simulink model "agws_fastTT"  (R2016a)
settings: Solver=ode4  StartTime=0.0  StopTime=1  FixedStep=Ts  RelTol=1e-3
values from neighbouring files (symbols this model uses):
  M1_BeMo_d = zeros(7,M1_n_mode)    [AcO_Ctrl_headless_cfg.m]    (also in agws_cfg.m = 1e-6*bsxfun(@times,randn(7,M1_n_mode),scale); agws_fastTT_cfg.m = 1e-6*bsxfun(@times,randn(7,M1_n_mode),scale))
  M1_RiBo_d = zeros(7,6)    [AcO_Ctrl_headless_cfg.m]    (also in agws_cfg.m = [M1_Txyz0 M1_Rxyz0]; agws_fastTT_cfg.m = [M1_Txyz0 M1_Rxyz0])
  M2_RiBo_d = zeros(7,6)    [AcO_Ctrl_headless_cfg.m]    (also in agws_cfg.m = [M2_Txyz0 M2_Rxyz0]; agws_fastTT_cfg.m = [M2_Txyz0 M2_Rxyz0])
  Ts = 1/fs    (= 0.002)    [AcO_Ctrl_headless_cfg.m]    (also in agws_fastTT_cfg.m = 0.005)
undefined symbols (not defined in the file or in its folder): R
libraries: CEO x4
settings Model: Creator=rconan  LastModifiedBy=rconan
settings DataIOCC: LimitDataPoints=on  SaveFormat=Array
settings HardwareCC: ProdBitPerPointer=32  ProdLargestAtomicFloat=None  ProdIntDivRoundTo=Undefined  ProdEndianess=Unspecified  ProdWordSize=32  ProdHWDeviceType=32-bit Generic
settings ModelReferenceCC: PropagateSignalLabelsOutOfModel=off
settings ConfigComp: CovModelRefEnable=Off

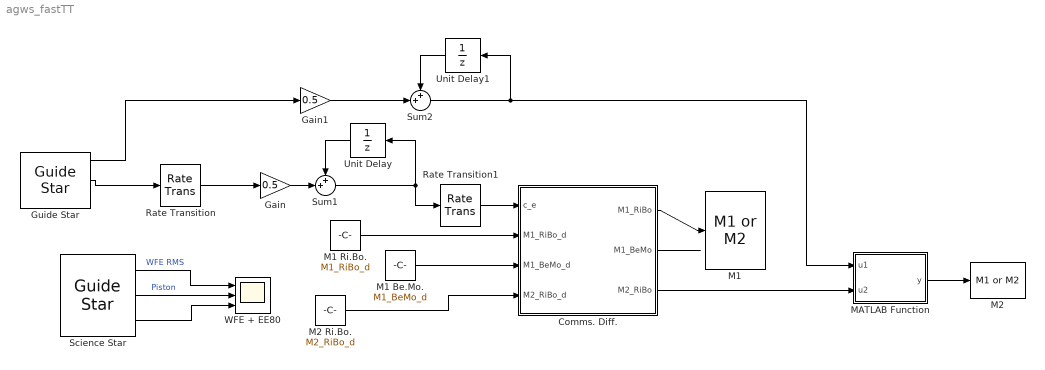
== system agws_fastTT ==
  Comms. Diff. : MATLAB Function  TreatAsAtomicUnit=on
  Gain : Gain  Gain=0.5
  Gain1 : Gain  Gain=0.5
  Guide Star : CEO/Guide Star  zenith=gs_zen  azimuth=gs_azi  photometry=R - 0.640  magnitude=0  rays_origin=[0,0,25]  rays_box_size=25.5  rays_box_sampling=16  sensor=GeometricShackHartmann  sampleTime=[Ts,0]  n_lenslet=30  d=26/30  n_cam=128  px_scale=NaN  intensity_threshold=0.2  a=1  b=1  wfe_rms=off  piston=off  segment_piston=off  ee80=off  sens=off  calibration_file=[upper(gcs),'_Calibration']  coms=gs_calib  coms_size=gs_calib_size  svd_truncation=[0,6]
  M1 : CEO/M1 or M2  mirror=M1  TxyzRxyz=on  mode_coefs=on  n_mode=42  sampleTime=[-1,0]
  M1 Be.Mo. : Constant  Value=M1_BeMo_d
  M1 Ri.Bo. : Constant  Value=M1_RiBo_d
  M2 : CEO/M1 or M2  mirror=M2  TxyzRxyz=on  mode_coefs=off  n_mode=66  sampleTime=[-1,0]
  M2 Ri.Bo. : Constant  Value=M2_RiBo_d
  MATLAB Function : MATLAB Function  TreatAsAtomicUnit=on
  Rate Transition : RateTransition  OutPortSampleTime=M1_Ts
  Rate Transition1 : RateTransition  OutPortSampleTime=Ts
  Science Star : CEO/Guide Star  zenith=0  azimuth=0  photometry=R - 0.640  magnitude=0  rays_origin=[0,0,25]  rays_box_size=25.5  rays_box_sampling=256  sensor=Imaging  sampleTime=[Ts,0]  n_lenslet=1  d=26  n_cam=128  px_scale=0.00127  intensity_threshold=0.5  a=2  b=1  wfe_rms=on  piston=off  segment_piston=on  ee80=on  sens=off  calibration_file=[]  coms=[]  coms_size=14  svd_truncation=0
  Sum1 : Sum  Inputs=++|
  Sum2 : Sum  Inputs=++|
  Unit Delay : UnitDelay  SampleTime=-1
  Unit Delay1 : UnitDelay  SampleTime=-1
  WFE + EE80 : Scope  NumInputPorts=3
  wires:
  Gain/1 -> Sum1/2
  Sum1/1 -> Rate Transition1/1, Unit Delay/1
  Unit Delay/1 -> Sum1/1
  Science Star/1 -> WFE + EE80/1  "WFE RMS"
  M1 Ri.Bo./1 -> Comms. Diff./2(M1_RiBo_d)
  Comms. Diff./1(M1_RiBo) -> M1/1
  Science Star/2 -> WFE + EE80/2  "Piston"
  Science Star/3 -> WFE + EE80/3
  Comms. Diff./2(M1_BeMo) -> ?
  M2 Ri.Bo./1 -> Comms. Diff./4(M2_RiBo_d)
  M1 Be.Mo./1 -> Comms. Diff./3(M1_BeMo_d)
  Guide Star/2 -> Rate Transition/1
  Rate Transition/1 -> Gain/1
  Rate Transition1/1 -> Comms. Diff./1(c_e)
  Gain1/1 -> Sum2/2
  Sum2/1 -> MATLAB Function/1(u1), Unit Delay1/1
  Unit Delay1/1 -> Sum2/1
  Guide Star/1 -> Gain1/1
  Comms. Diff./3(M2_RiBo) -> MATLAB Function/2(u2)
  MATLAB Function/1(y) -> M2/1

== matlab function agws_fastTT/MATLAB Function ==
  data: u1 input; y output; u2 input
function y = removeTT(u1,u2)
%#codegen

y = u2;
y(:,4:5) = u2(:,4:5) - reshape(u1,2,7)';

== matlab function agws_fastTT/Comms. Diff. ==
  data: c_e input; M1_RiBo output; M1_RiBo_d input; M1_BeMo output; M1_BeMo_d input; M2_RiBo output; M2_RiBo_d input
function [M1_RiBo,M1_BeMo,M2_RiBo]= diff(c_e,M1_RiBo_d,M1_BeMo_d,M2_RiBo_d)
%#codegen

M1_Txyz = zeros(1,21);
M1_Rxyz = zeros(1,21);
M2_Rxyz = zeros(1,21);

M1_Rxyz(1:20) = c_e(1:20);
M2_Rxyz(1:20) = c_e(21:40);
M1_Txyz(1:20) = c_e(41:60);
M2_Txyz       = c_e(61:81);

M1_TR = [ reshape(M1_Txyz,3,7) ; reshape(M1_Rxyz,3,7) ];
%M1_TR = reshape( M1_TR, 1 , 42);

M2_TR = [ reshape(M2_Txyz,3,7) ; reshape(M2_Rxyz,3,7) ];
%M2_TR = reshape( M2_TR, 1 , 42);

M1_RiBo = M1_RiBo_d - M1_TR';
M2_RiBo = M2_RiBo_d - M2_TR';

M1_BeMo = M1_BeMo_d - reshape(c_e(82:end),[],7)';
